simulink model "MPCS_2D_Formulation"  (R2016a)
settings: Solver=FixedStepDiscrete  StartTime=0.0  StopTime=Inf  FixedStep=Tmpc  RelTol=1e-3
InitFcn:
  | Tmpc = 1/1000;
libraries: slrtlib x5
settings Model: SimulationMode=external  ExplicitPartitioning=on  Creator=The MathWorks, Inc.  LastModifiedBy=SLRT
settings SolverCC: EnableConcurrentExecution=on
settings DataIOCC: SaveFinalState=on  SaveFormat=StructureWithTime
settings OptimizationCC: BlockReduction=off  OptimizeBlockIOStorage=off  BufferReuse=off  GlobalBufferReuse=off  ExpressionFolding=off  ExpressionDepthLimit=2147483647  LocalBlockOutputs=off
settings DebuggingCC: ReadBeforeWriteMsg=DisableAll  WriteAfterWriteMsg=DisableAll  WriteAfterReadMsg=DisableAll  UnderspecifiedInitializationDetection=Classic  MergeDetectMultiDrivingBlocksExec=none  SolverPrmCheckMsg=warning  InheritedTsInSrcMsg=none  FcnCallInpInsideContextMsg=EnableAllAsWarning  StateNameClashWarn=warning
settings HardwareCC: ProdBitPerPointer=32  ProdLargestAtomicFloat=None  ProdWordSize=32  ProdHWDeviceType=Generic->32-bit x86 compatible
settings ModelReferenceCC: PropagateSignalLabelsOutOfModel=off
settings RTWCC: SystemTargetFile=slrt.tlc  TLCOptions=-axPCMaxOverloads=100000 -axPCOverLoadLen=100000 -axPCStartupFlag=5  TemplateMakefile=slrt_default_tmf  Description=Simulink Real-Time  RTWVerbose=off  RTWCompilerOptimization=on
settings RTWCC: CustomInclude=|
  | C:\Users\SLRT\Desktop\Swift\include
  | C:\Users\SLRT\Desktop\Swift\ldl\include
settings RTWCC: CustomSource=|
  | C:\Users\SLRT\Desktop\Swift\ldl\src\ldl.c
  | C:\Users\SLRT\Desktop\Swift\src\Auxilary.c
  | C:\Users\SLRT\Desktop\Swift\src\Prime.c
  | C:\Users\SLRT\Desktop\Swift\src\timer.c
settings SimulinkRealTimeCC: GeneratePreprocessorConditionals=Disable all  RL32LogBufSizeModifier=38000000  xPCRL32EventNumber=50000000  xPCisModelTimeout=off  xPCModelTimeoutSecs=20  xPCConcurrentTasks=on
settings ConfigComp: CovSFcnEnable=off
settings SimscapeCC: SelectedTab=General

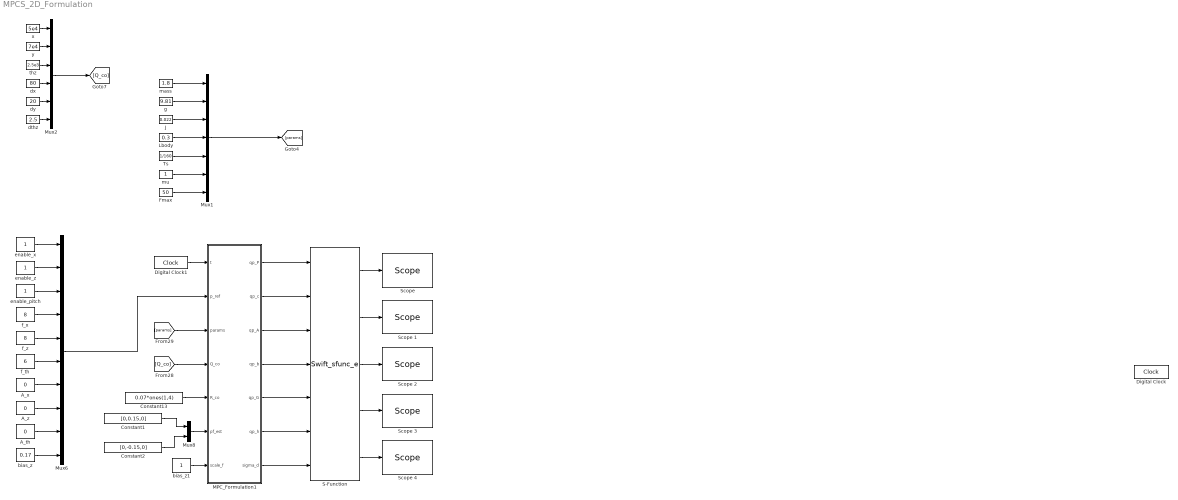
== system MPCS_2D_Formulation ==
  A_th : Constant  Value=0  SampleTime=Tmpc
  A_x : Constant  Value=0  SampleTime=Tmpc
  A_z : Constant  Value=0  SampleTime=Tmpc
  Constant1 : Constant  Value=[0,0.15,0]  SampleTime=Tmpc
  Constant13 : Constant  Value=0.07*ones(1,4)  SampleTime=Tmpc
  Constant2 : Constant  Value=[0,-0.15,0]  SampleTime=Tmpc
  Digital Clock1 : DigitalClock  SampleTime=Tmpc
  Fmax : Constant  Value=50  SampleTime=Tmpc
  J : Constant  Value=0.022  SampleTime=Tmpc
  Lbody : Constant  Value=0.3  SampleTime=Tmpc
  MPC_Formulation1 : MATLAB Function  TreatAsAtomicUnit=on  SystemSampleTime=Tmpc
  Mux1 : Mux  Inputs=7
  Mux2 : Mux  Inputs=6
  Mux6 : Mux  Inputs=10
  Mux8 : Mux  Inputs=2
  S-Function : S-Function  FunctionName=Swift_sfunc_e  SFunctionDeploymentMode=off  EnableBusSupport=off
  "Scope " : slrtlib/Displays and Logging/Scope   scopeno=1  scopetype=Target  autostart=on  viewmode=Numerical  formatstr='%15.6f'  grid=on  ylimits=[0,0]  nosamples=3  noprepostsamples=0  interleave=1  triggermode=FreeRun  triggersignal=1  trigsignalfromport=off  triggerlevel=0.0  triggerslope=Either  triggerscope=1  triggersample=0  filename=data.dat  mode=Lazy  writesize=512  autorestart=off  dynamicfilemode=off  maxwritefilesize=512*1024^2
  Scope 1 : slrtlib/Displays and Logging/Scope   scopeno=2  scopetype=Target  autostart=on  viewmode=Numerical  formatstr='%15.6f'  grid=on  ylimits=[0,0]  nosamples=3  noprepostsamples=0  interleave=1  triggermode=FreeRun  triggersignal=1  trigsignalfromport=off  triggerlevel=0.0  triggerslope=Either  triggerscope=1  triggersample=0  filename=data.dat  mode=Lazy  writesize=512  autorestart=off  dynamicfilemode=off  maxwritefilesize=512*1024^2
  Scope 2 : slrtlib/Displays and Logging/Scope   scopeno=3  scopetype=Target  autostart=on  viewmode=Numerical  formatstr='%15.6f'  grid=on  ylimits=[0,0]  nosamples=3  noprepostsamples=0  interleave=1  triggermode=FreeRun  triggersignal=1  trigsignalfromport=off  triggerlevel=0.0  triggerslope=Either  triggerscope=1  triggersample=0  filename=data.dat  mode=Lazy  writesize=512  autorestart=off  dynamicfilemode=off  maxwritefilesize=512*1024^2
  Scope 3 : slrtlib/Displays and Logging/Scope   scopeno=4  scopetype=Target  autostart=on  viewmode=Graphical redraw  formatstr='%15.6f'  grid=on  ylimits=[0,0]  nosamples=250  noprepostsamples=0  interleave=1  triggermode=FreeRun  triggersignal=1  trigsignalfromport=off  triggerlevel=0.0  triggerslope=Either  triggerscope=1  triggersample=0  filename=data.dat  mode=Lazy  writesize=512  autorestart=off  dynamicfilemode=off  maxwritefilesize=512*1024^2
  Scope 4 : slrtlib/Displays and Logging/Scope   scopeno=5  scopetype=Target  autostart=on  viewmode=Numerical  formatstr='%15.6f'  grid=on  ylimits=[0,0]  nosamples=3  noprepostsamples=0  interleave=1  triggermode=FreeRun  triggersignal=1  trigsignalfromport=off  triggerlevel=0.0  triggerslope=Either  triggerscope=1  triggersample=0  filename=data.dat  mode=Lazy  writesize=512  autorestart=off  dynamicfilemode=off  maxwritefilesize=512*1024^2
  Ts : Constant  Value=1/160  SampleTime=Tmpc
  bias_z : Constant  Value=0.17  SampleTime=Tmpc
  bias_z1 : Constant  SampleTime=Tmpc
  dthz : Constant  Value=2.5  SampleTime=Tmpc
  dx : Constant  Value=80  SampleTime=Tmpc
  dy : Constant  Value=20  SampleTime=Tmpc
  enable_pitch : Constant  SampleTime=Tmpc
  enable_x : Constant  SampleTime=Tmpc
  enable_z : Constant  SampleTime=Tmpc
  f_th : Constant  Value=6  SampleTime=Tmpc
  f_x : Constant  Value=8  SampleTime=Tmpc
  f_z : Constant  Value=8  SampleTime=Tmpc
  g : Constant  Value=9.81  SampleTime=Tmpc
  mass : Constant  Value=1.8  SampleTime=Tmpc
  mu : Constant  SampleTime=Tmpc
  thz : Constant  Value=2.5e3  SampleTime=Tmpc
  x : Constant  Value=5e4  SampleTime=Tmpc
  y : Constant  Value=7e4  SampleTime=Tmpc
  Digital Clock : DigitalClock  IOType=siggen
  wires:
  Constant13/1 -> MPC_Formulation1/5(R_co)
  [params] -> MPC_Formulation1/3(params)
  [Q_co] -> MPC_Formulation1/4(Q_co)
  Constant1/1 -> Mux8/1
  Constant2/1 -> Mux8/2
  Mux8/1 -> MPC_Formulation1/6(pf_est)
  enable_x/1 -> Mux6/1
  enable_z/1 -> Mux6/2
  enable_pitch/1 -> Mux6/3
  f_x/1 -> Mux6/4
  f_z/1 -> Mux6/5
  bias_z/1 -> Mux6/10
  A_th/1 -> Mux6/9
  A_z/1 -> Mux6/8
  A_x/1 -> Mux6/7
  f_th/1 -> Mux6/6
  Mux6/1 -> MPC_Formulation1/2(p_ref)
  bias_z1/1 -> MPC_Formulation1/7(scale_f)
  MPC_Formulation1/1(qp_P) -> S-Function/1
  MPC_Formulation1/2(qp_c) -> S-Function/2
  MPC_Formulation1/3(qp_A) -> S-Function/3
  MPC_Formulation1/4(qp_b) -> S-Function/4
  MPC_Formulation1/5(qp_G) -> S-Function/5
  MPC_Formulation1/6(qp_h) -> S-Function/6
  MPC_Formulation1/7(sigma_d) -> S-Function/7
  S-Function/1 -> "Scope "/1
  S-Function/2 -> Scope 1/1
  S-Function/3 -> Scope 2/1
  S-Function/4 -> Scope 3/1
  S-Function/5 -> Scope 4/1
  Digital Clock1/1 -> MPC_Formulation1/1(t)
  Mux2/1 -> [Q_co]
  x/1 -> Mux2/1
  y/1 -> Mux2/2
  thz/1 -> Mux2/3
  dx/1 -> Mux2/4
  dy/1 -> Mux2/5
  dthz/1 -> Mux2/6
  mass/1 -> Mux1/1
  g/1 -> Mux1/2
  J/1 -> Mux1/3
  Lbody/1 -> Mux1/4
  Ts/1 -> Mux1/5
  Mux1/1 -> [params]
  mu/1 -> Mux1/6
  Fmax/1 -> Mux1/7

== matlab function MPCS_2D_Formulation/MPC_Formulation1 ==
  data: t input; p_ref input; qp_P output; qp_c output; qp_A output; qp_b output; qp_G output; qp_h output; sigma_d output; params input; Q_co input; R_co input; pf_est input; scale_f input
function [qp_P,qp_c,qp_A,qp_b,qp_G,qp_h,sigma_d]  = ...
fcn(t,p_ref,params,Q_co,R_co,pf_est,scale_f)

X_op = rand(6,1);  
u_op = rand(4,1);

% parameters
mass = params(1);
g = params(2);
J = params(3);
L = params(4);
Tmpc = params(5);
mu = params(6);
Fmax = params(7);
sigma_d = 0;

% reference trajectory
enable_x = p_ref(1);
enable_z = p_ref(2);
enable_th = p_ref(3);
f_x = p_ref(4);
f_z = p_ref(5);
f_th = p_ref(6);
A_x = p_ref(7);
A_z = p_ref(8);
A_th = p_ref(9);
bias_z = p_ref(10);

% desired state
x_d = A_x * sin(f_x * t);
z_d = A_z * sin(f_z * t) + bias_z;
th_d = A_th * sin(f_th * t);

dx_d = A_x * f_x * cos(f_x * t);
dz_d = A_z * f_z * cos(f_z * t);
dth_d = A_th * f_th * cos(f_th * t);

Xr = [x_d,z_d,th_d,dx_d,dz_d,dth_d]';


% params for MPC
k = 7;
Nx = 6;
Nu = 4;
Nux = Nx + Nu;

% foot position
p1 = [pf_est(1);pf_est(3)];  % left foot
p2 = [pf_est(4);pf_est(6)];  % right foot

p.mass = mass;
p.g = g;
p.J = J;
p.p1 = p1;
p.p2 = p2;

ur = [0;mass*g/2;0;mass*g/2];

% final desired state
t_f = t + k * Tmpc;
x_d = A_x * sin(f_x * t_f);
z_d = A_z * sin(f_z * t_f) + bias_z;
th_d = A_th * sin(f_th * t_f);

dx_d = A_x * f_x * cos(f_x * t_f);
dz_d = A_z * f_z * cos(f_z * t_f);
dth_d = A_th * f_th * cos(f_th * t_f);

Xr_f = [x_d,z_d,th_d,dx_d,dz_d,dth_d]';

%%
Q = diag(Q_co); % state weight
R = diag(R_co); % control weight    

% vectors
% qq = Q * (X_op - Xr);
rr = R * (u_op - ur);

% final state
Qf = scale_f * Q;
qf = Qf * (X_op - Xr);

% --- continuous system ---
% state: dX = [dx;dth;Ddx;Ddth]
% control: du = [dF1;dF2]
% DdX = Ac * dX + Bc * du + Dc
Ac = zeros(Nx);
Ac(1:Nx/2,Nx/2+1:Nx) = eye(Nx/2);
Ac(Nx,1:2) = 1/J * (hatMap1(u_op(1:2)) + hatMap1(u_op(3:4)));

% control du = [dF1;dF2]
Bc = zeros(6,4);
Bc(4:5,1:4) = 1/mass * [1,0,1,0;0,1,0,1];
x_op = X_op(1:2);
Bc(6,1:4) = 1/J * [hatMap1(p1 - x_op),hatMap1(p2 - x_op)];

% constant term
Dc = dyn_nonlin1(X_op,u_op,p);

% --- discrete system ---
% Ad = eye(Nx) + Tmpc * Ac;
Ad = expm(Ac * Tmpc);
Bd = Tmpc * Bc;
Dd = Tmpc * Dc;

%% MPC: QP
% prelocation
% min. z' * H * z + vg' * z
len_z = Nux * k;
H = zeros(len_z , len_z);
H(1:Nu , 1:Nu) = R;
idx_Qf = len_z - Nx + 1 : len_z;
H(idx_Qf, idx_Qf) = Qf;

vg = zeros(len_z,1);
vg(1:Nu,1) = rr;
vg(Nux-Nx+1 : Nux , 1) = qf;

% P * z <= h
P = zeros(Nu * k, len_z);
Fu = [1 -mu;-1 -mu];
Fu = [Fu,zeros(2);zeros(2),Fu];
P(1:Nu,1:Nu) = Fu;

% C * z == b
C = zeros(Nx*k,len_z);
C(1:Nx,1:Nux) = [-Bd, eye(Nx)];

b = zeros(Nx * k,1);
b(1:Nx,1) = Ad * zeros(Nx,1) + Dd;

% lb <= z <= ub
umin = [-mu*Fmax;0;-mu*Fmax;0];
umax = [mu*Fmax;Fmax;mu*Fmax;Fmax];

% Xmin = [-0.4;0;-3;...
%     -10;-10;-50];
% Xmax = [0.4;1;3;...
%         10;10;50];
Xmin = -Inf * ones(6,1);
Xmax = Inf * ones(6,1);

ub = zeros(len_z,1);
ub(1:Nu,1) = [umax - u_op];
ub(len_z-Nx+1 : len_z , 1) = Xmax - X_op;

lb = zeros(len_z,1);
lb(1:Nu,1) = [umin - u_op];
lb(len_z-Nx+1 : len_z , 1) = Xmin - X_op;

h_op = zeros(len_z,1);
h_op(1:Nu,1) = u_op;
h_op(len_z-Nx+1 : len_z , 1) = X_op;

for ii = 1:k-1
    %% quadratic cost
    idx_H = Nu + (ii-1) * Nux + (1:Nux);
    H_new = [Q, zeros(Nx,Nu);zeros(Nu,Nx),R];
    H(idx_H,idx_H) = H_new;
    
    % desired statet
    t_i = t + ii * Tmpc;
    x_d = enable_x * A_x * sin(f_x * t_i);
    z_d = enable_z * A_z * sin(f_z * t_i) + bias_z;
    th_d = enable_th * A_th * sin(f_th * t_i);

    dx_d = enable_x * A_x * f_x * cos(f_x * t_i);
    dz_d = enable_z * A_z * f_z * cos(f_z * t_i);
    dth_d = enable_th * A_th * f_th * cos(f_th * t_i);

    Xr_i = [x_d,z_d,th_d,dx_d,dz_d,dth_d]';
    
    qq = Q * (X_op - Xr_i);

    idx_g = Nu + (ii-1) * Nux + (1:Nux);
    vg(idx_g,1) = [qq;rr];
    
    %% inequality constraints
    idx_Fu1 = Nu + (ii-1) * Nu + (1:Nu);
    idx_Fu2 = Nux + (ii-1) * Nux + (1:Nu);
    P(idx_Fu1,idx_Fu2) = Fu;

    % equality constraint for linear dynamics
    idx_C1 = Nx + (ii-1) * Nx + (1:Nx);
    idx_C2 = Nu + (ii-1) * Nux + (1:(Nux + Nx));    
    C(idx_C1,idx_C2) = [-Ad, -Bd, eye(Nx)];

    idx_b = Nx + (ii-1) * Nx + (1:Nx);
    b(idx_b,1) = Dd;
    
    % bound on state
    idx_zbound = Nu + (ii-1) * Nux + (1:Nux);
    lb(idx_zbound,1) = [Xmin-X_op;umin-u_op];
    ub(idx_zbound,1) = [Xmax-X_op;umax-u_op];
    
    h_op(idx_zbound,1) = [X_op;u_op];

end

h = -P * h_op;

qp_P = H(:);
qp_c = vg;
qp_A = C(:);
qp_b = b;
qp_G = P(:);
qp_h = h;

e = X_op - Xr;

end

function Mv = hatMap1(v)

Mv = [v(2), -v(1)];

end

function dXdt = dyn_nonlin1(X,u,p)
% simulink
mass = p.mass;
g = p.g;
J = p.J;
p1 = p.p1;
p2 = p.p2;

x = X(1);
z = X(2);

F1 = u(1:2);
F2 = u(3:4);

pCOM = [x;z];
r1 = p1 - pCOM;
r2 = p2 - pCOM;
tau = hatMap1(r1) * F1 + hatMap1(r2) * F2;

ddx = (F1(1) + F2(1)) / mass;
ddz = (F1(2) + F2(2)) / mass - g;
ddth = tau / J;

dXdt = zeros(6,1);
dXdt(1:3) = X(4:6);
dXdt(4:6) = [ddx ddz ddth]';

end
